simulink model "sigma_delta_adc"  (R2022a)
settings: Solver=VariableStepAuto  StartTime=0.0  StopTime=0.1  RelTol=1e-3
values from neighbouring files (symbols this model uses):
  amp = 0.25    [run_adc.m]
  ff = 0.1e3    (= 100)    [run_adc.m]
  ts = 1/fs    (= 9.765625e-07)    [run_adc.m]
settings Model: Creator=NINGMEI  LastModifiedBy=NINGMEI
settings DataIOCC: ReturnWorkspaceOutputs=off  LoggingToFile=on  LoggingFileName=adc_out.mat
settings ModelReferenceCC: EnableRefExpFcnMdlSchedulingChecks=off
settings RTWCC: Description=Generic Real-Time Target

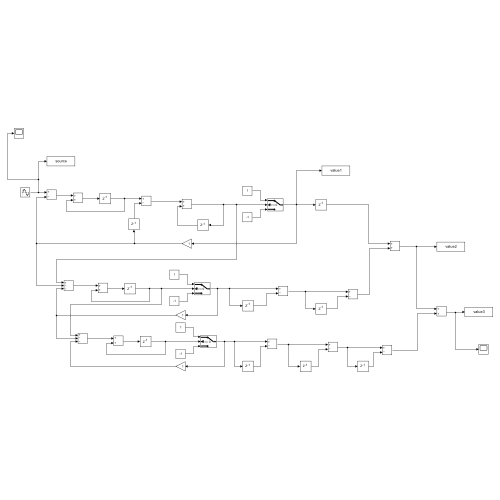
[thumbnail: Simulink's stored preview of the top-level diagram]
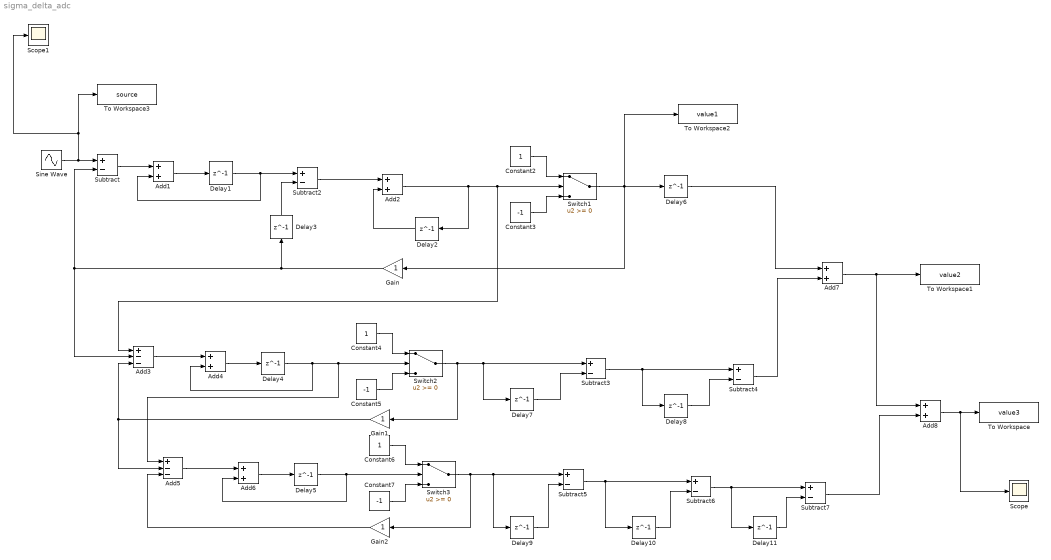
== system sigma_delta_adc ==
  Add{1..2,4,6..8} (6 alike) : Sum
  Add3 : Sum  Inputs=+--
  Add5 : Sum  Inputs=+--
  Constant2 : Constant
  Constant3 : Constant  Value=-1
  Constant4 : Constant
  Constant5 : Constant  Value=-1
  Constant6 : Constant
  Constant7 : Constant  Value=-1
  Delay{1..11} (11 alike) : Delay  DelayLength=1  InitialCondition=0
  Gain : Gain
  Gain1 : Gain
  Gain2 : Gain
  Scope : Scope
  Scope1 : Scope
  Sine Wave : Sin  Amplitude=amp  Frequency=2*pi*ff  SampleTime=ts
  Subtract{,2..7} (7 alike) : Sum  Inputs=+-
  Switch1 : Switch  SaturateOnIntegerOverflow=off  InputSameDT=off
  Switch2 : Switch  SaturateOnIntegerOverflow=off  InputSameDT=off
  Switch3 : Switch  SaturateOnIntegerOverflow=off  InputSameDT=off
  To Workspace : ToWorkspace  VariableName=value3  SampleTime=-1
      settings: Save2DSignal=2-D array (concatenate along first dimension)
  To Workspace1 : ToWorkspace  VariableName=value2  SampleTime=-1
      settings: Save2DSignal=2-D array (concatenate along first dimension)
  To Workspace2 : ToWorkspace  VariableName=value1  SampleTime=-1
      settings: Save2DSignal=2-D array (concatenate along first dimension)
  To Workspace3 : ToWorkspace  VariableName=source  SampleTime=-1
      settings: Save2DSignal=2-D array (concatenate along first dimension)
  wires:
  Sine Wave/1 -> Scope1/1, To Workspace3/1, Subtract/1
  Subtract/1 -> Add1/1
  Constant3/1 -> Switch1/3
  Constant2/1 -> Switch1/1
  Add1/1 -> Delay1/1
  Delay3/1 -> Subtract2/2
  Delay1/1 -> Add1/2, Subtract2/1
  Subtract2/1 -> Add2/1
  Delay2/1 -> Add2/2
  Switch1/1 -> Gain/1, To Workspace2/1, Delay6/1
  Add2/1 -> Switch1/2, Add3/1, Delay2/1
  Add3/1 -> Add4/1
  Add4/1 -> Delay4/1
  Delay4/1 -> Add5/1, Switch2/2, Add4/2
  Constant5/1 -> Switch2/3
  Constant4/1 -> Switch2/1
  Gain/1 -> Delay3/1, Subtract/2, Add3/2
  Switch2/1 -> Gain1/1, Delay7/1, Subtract3/1
  Gain1/1 -> Add5/2, Add3/3
  Delay5/1 -> Add6/2, Switch3/2
  Add6/1 -> Delay5/1
  Add5/1 -> Add6/1
  Constant7/1 -> Switch3/3
  Constant6/1 -> Switch3/1
  Switch3/1 -> Delay9/1, Subtract5/1, Gain2/1
  Gain2/1 -> Add5/3
  Delay7/1 -> Subtract3/2
  Delay8/1 -> Subtract4/2
  Subtract3/1 -> Delay8/1, Subtract4/1
  Delay6/1 -> Add7/1
  Subtract4/1 -> Add7/2
  Delay9/1 -> Subtract5/2
  Subtract5/1 -> Delay10/1, Subtract6/1
  Delay10/1 -> Subtract6/2
  Subtract6/1 -> Delay11/1, Subtract7/1
  Delay11/1 -> Subtract7/2
  Subtract7/1 -> Add8/2
  Add7/1 -> To Workspace1/1, Add8/1
  Add8/1 -> Scope/1, To Workspace/1
